simulink model "stellaris_test_gpio_xpc"  (R2012b)
settings: Solver=FixedStepDiscrete  StartTime=0.0  StopTime=inf  FixedStep=0.001  RelTol=1e-3
libraries: xpclib x3, speedgoatlib_IO101 x2
settings Model: BufferReuse=off  Creator=peselnikmg  LastModifiedBy=peselnikmg
settings DataIOCC: SignalLoggingSaveFormat=ModelDataLogs
settings OptimizationCC: BlockReduction=off  OptimizeBlockIOStorage=off  BufferReuse=off  ExpressionFolding=off  LocalBlockOutputs=off
settings HardwareCC: ProdIntDivRoundTo=Zero  ProdEndianess=LittleEndian  ProdHWDeviceType=Generic->32-bit x86 compatible
settings RTWCC: SystemTargetFile=xpctarget.tlc  TemplateMakefile=xpc_default_tmf  Description=xPC Target  ProcessScript=xpctarget_make_rtw_hook  RTWCompilerOptimization=On
settings xpcTargetCC: TargetFcnLib=ansi_tfl_table_tmw.mat  CodeReplacementLibrary=XPC_BLAS  ParMdlRefBuildCompliant=on  ConcurrentExecutionCompliant=on  CombineSignalStateStructs=off  GRTInterface=on  xPCTaskExecutionProfile=off  xPCRL32EventNumber=5000  xPCLoadParamSetFile=off  xPCConcurrentTasks=off  xPCEnableSFAnimation=off

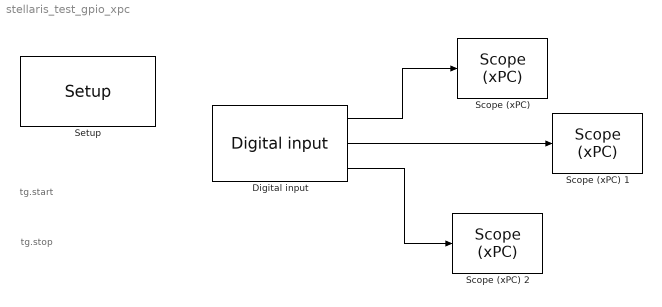
== system stellaris_test_gpio_xpc ==
  note: tg.start
  note: tg.stop
  Digital input : speedgoatlib_IO101/Digital input  id=1  groupChannel=Lower  lowerChannel=[1,2,3]  upperChannel=1  lowerDIDebounce=[0,0,0]  upperDIDebounce=0  ts=0.001  pciSlot=-1
  "Scope (xPC) " : xpclib/Misc./Scope (xPC)   scopeno=1  scopetype=Target  autostart=on  viewmode=Graphical redraw  formatstr='%15.6f'  grid=on  ylimits=[0,0]  nosamples=600  noprepostsamples=-50  interleave=1  triggermode=Signal triggering  triggersignal=1  triggerlevel=0.5  triggerslope=Rising  triggerscope=1  triggersample=0  filename=data.dat  mode=Lazy  writesize=512  autorestart=off  dynamicfilemode=off  maxwritefilesize=512*1024^2
  Scope (xPC) 1 : xpclib/Misc./Scope (xPC)   scopeno=2  scopetype=Target  autostart=on  viewmode=Graphical redraw  formatstr='%15.6f'  grid=on  ylimits=[0,0]  nosamples=600  noprepostsamples=-50  interleave=1  triggermode=Scope triggering  triggersignal=1  triggerlevel=0  triggerslope=Either  triggerscope=1  triggersample=0  filename=data.dat  mode=Lazy  writesize=512  autorestart=off  dynamicfilemode=off  maxwritefilesize=512*1024^2
  Scope (xPC) 2 : xpclib/Misc./Scope (xPC)   scopeno=3  scopetype=Target  autostart=on  viewmode=Graphical redraw  formatstr='%15.6f'  grid=on  ylimits=[0,0]  nosamples=600  noprepostsamples=-50  interleave=1  triggermode=Scope triggering  triggersignal=1  triggerlevel=0  triggerslope=Either  triggerscope=1  triggersample=0  filename=data.dat  mode=Lazy  writesize=512  autorestart=off  dynamicfilemode=off  maxwritefilesize=512*1024^2
  Setup : speedgoatlib_IO101/Setup  group=Digital setup lower channel  id=1  pciSlot=-1  adStartChannel=1  adNumChannel=32  adCoupling=Single-ended  adRange=-10 .. 10 Volts  adAcqMode=Standard  daChannel=[1:8]  daReset=[1]  daInitValue=[0]  lowerChannel=1:3  lowerDirection=Input  lowerDIDebounce=0  lowerDOReset=[1]  lowerDOInitValues=[0]  upperChannel=1  upperDirection=Output  upperDIDebounce=0  upperDOReset=0  upperDOInitValues=0
  wires:
  Digital input/2 -> Scope (xPC) 1/1
  Digital input/1 -> "Scope (xPC) "/1
  Digital input/3 -> Scope (xPC) 2/1
